simulink model "ANFISgain_tuning_simulink"  (R2024b)
settings: Solver=FixedStepAuto  StartTime=0.0  StopTime=1000  FixedStep=0.015  RelTol=1e-3
undefined symbols (not defined in the file or in its folder): sigbuilder_block, w_0
libraries: fuzblock x2, slpidlib x1, cstblocks x1
settings Model: Creator=bavejr  LastModifiedBy=lenovo pc
settings DebuggingCC: UnconnectedInputMsg=warning  UnconnectedOutputMsg=warning  UnconnectedLineMsg=warning
settings ModelReferenceCC: EnableRefExpFcnMdlSchedulingChecks=on
settings RTWCC: GPUComputeCapability=3.5  DLArmComputeVersion=19.05

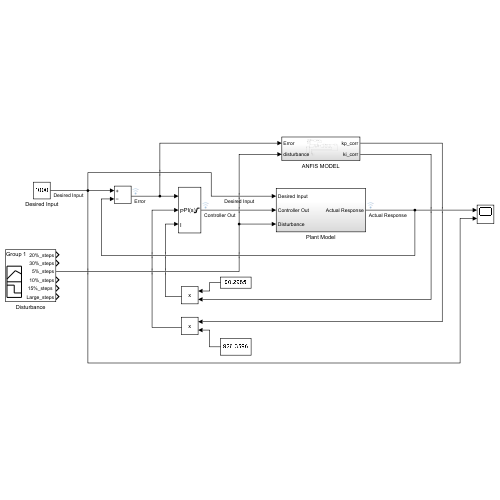
[thumbnail: Simulink's stored preview of the top-level diagram]
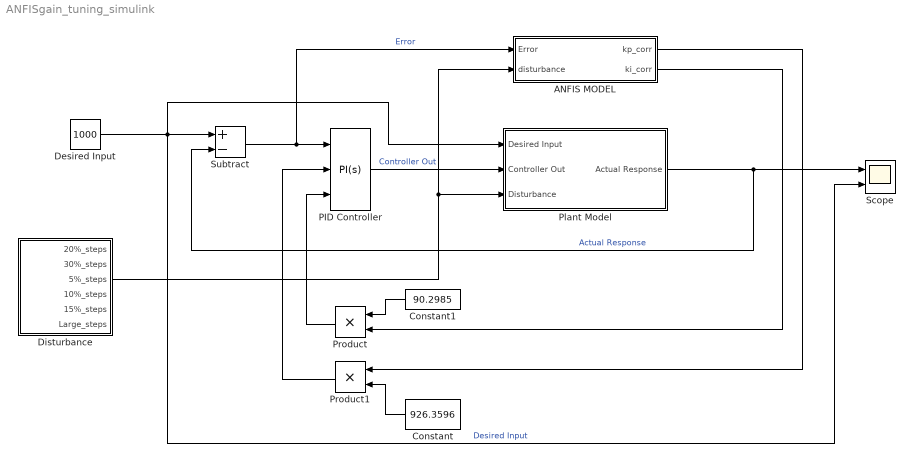
== system ANFISgain_tuning_simulink ==
  ANFIS MODEL : Subsystem
  Constant : Constant  Value=926.3596
  Constant1 : Constant  Value=90.2985
  Desired Input : Constant  Value=1000
  Disturbance : Subsystem  Tag=STV Subsys  LoadFcn=sigbuilder_block('load');  StartFcn=sigbuilder_block('start');  StopFcn=sigbuilder_block('stop');  ClipboardFcn=sigbuilder_block('clipboard');  mask(Sigbuilder block){tuvar=[0:10]}
      mask help: Simulink:masks:SigbuilderBlock_MD
      mask init:
      | if ~strcmp(get_param(bdroot(gcbh),'SimulationStatus'),'stopped') tuvar = sigbuilder_block('maskInit'); end
      settings: CopyFcn=sigbuilder_block('copy');  DeleteFcn=sigbuilder_block('delete');  ModelCloseFcn=sigbuilder_block('modelClose');  PreSaveFcn=sigbuilder_block('preSave');  PauseFcn=sigbuilder_block('pause');  ContinueFcn=sigbuilder_block('continue');  NameChangeFcn=sigbuilder_block('namechange');  OpenFcn=sigbuilder_block('open',[5.5 5.5 949 474.5 ]);  CloseFcn=sigbuilder_block('close');
      mask Display: plot(0, 0, 100, 100,[2, 2, 32, 32, 2], [68, 8, 8, 68, 68],[32, 2], [38, 38], [32, 19, 2],[53, 60, 44], [32, 17, 17, 2],[16, 16, 31, 31]);txt = getActiveGroup(gcbh);text(2, 100, txt,'verticalAlignment', 'top');
  PID Controller : slpidlib/PID Controller  Controller=PI  Form=Parallel  TimeDomain=Continuous-time  UseExternalTs=off  SampleTime=-1  IntegratorMethod=Forward Euler  FilterMethod=Forward Euler  ControllerParametersSource=external  P=8  I=2  UseKiTs=off  D=0  UseExternalDerivativeSource=off  N=100  UseFilter=on  TunerSelectOption=Frequency Response Based  InitialConditionSource=internal  InitialConditionForIntegrator=0.2  InitialConditionForFilter=0  DifferentiatorICPrevScaledInput=0  ExternalReset=none  TrackingMode=off  Kt=1  LimitOutput=on  SatLimitsSource=internal  UpperSaturationLimit=inf  LowerSaturationLimit=-inf  LinearizeAsGain=on  AntiWindupMode=back-calculation  Kb=0.0975  LimitIntegrator=off  UpperIntegratorSaturationLimit=inf  LowerIntegratorSaturationLimit=-inf  POutMin=[]  POutMax=[]  IOutMin=[]  IOutMax=[]  DOutMin=[]  DOutMax=[]  NOutMin=[]  NOutMax=[]  SumOutMin=[]  SumOutMax=[]  SaturationOutMin=[]  SaturationOutMax=[]  PParamMin=[]  PParamMax=[]  IParamMin=[]  IParamMax=[]  DParamMin=[]  DParamMax=[]  NParamMin=[]  NParamMax=[]  KbParamMin=[]  KbParamMax=[]  KtParamMin=[]  KtParamMax=[]  KbOutMin=[]  KbOutMax=[]  KtOutMin=[]  KtOutMax=[]  IntegratorOutMin=[]  IntegratorOutMax=[]  FilterOutMin=[]  FilterOutMax=[]  SumI1OutMin=[]  SumI1OutMax=[]  SumI2OutMin=[]  SumI2OutMax=[]  SumI3OutMin=[]  SumI3OutMax=[]  SumI4OutMin=[]  SumI4OutMax=[]  SumDOutMin=[]  SumDOutMax=[]  DifferentiatorOutMin=[]  DifferentiatorOutMax=[]  FilterDiffOutCoefMin=[]  FilterDiffOutCoefMax=[]  ReciprocalOutMin=[]  ReciprocalOutMax=[]  SumDenOutMin=[]  SumDenOutMax=[]  SumNumOutMin=[]  SumNumOutMax=[]  DivideOutMin=[]  DivideOutMax=[]  UdiffTsProdOutMin=[]  UdiffTsProdOutMax=[]  NTsProdOutMin=[]  NTsProdOutMax=[]  UintegralTsProdOutMin=[]  UintegralTsProdOutMax=[]  UngainTsProdOutMin=[]  UngainTsProdOutMax=[]  ClampingZeroOutDataTypeStr=Inherit: Inherit via back propagation  ClampingZeroOutMin=[]  ClampingZeroOutMax=[]  FilterDenConstantOutDataTypeStr=Inherit: Inherit via back propagation  FilterDenConstantOutMin=[]  FilterDenConstantOutMax=[]  PCopyOutDataTypeStr=Inherit: Inherit via back propagation  PCopyOutMin=[]  PCopyOutMax=[]  NCopyOutDataTypeStr=Inherit: Inherit via back propagation  NCopyOutMin=[]  NCopyOutMax=[]  IntegratorContinuousStateAttributes=''  IntegratorStateMustResolveToSignalObject=off  IntegratorRTWStateStorageClass=Auto  FilterContinuousStateAttributes=''  FilterStateMustResolveToSignalObject=off  FilterRTWStateStorageClass=Auto  ParallelPVariant=ExternalParameters  IdealPVariant=Disabled  IVariant=ExternalParameters  DVariant=Disabled  IntegratorVariant=Continuous  SatVariant=Enabled  AWVariant=BackCalculation  PCopyVariant=Disabled  TRVariant=Disabled  FdbkBlocksVariant=Forward  IdealPFdbkVariant=Disabled  SatFdbkVariant=Disabled  DerivativeFilterVariant=Disabled  NVariant=Disabled  NCopyVariant=Disabled_SignalSpec  FilterICVariant=Disabled  IntegratorICVariant=InternalICs  ExternalResetVariant=Disabled  TRSumVariant=Passthrough  SumFdbkVariant=Disabled  SumVariant=Sum_PI  TsampFilterVariant=InternalTs  TsampNgainVariant=Passthrough  TsampIntegralVariant=Disabled_SignalSpec  ExternalSaturationOutDataTypeStr=Inherit: Same as second input  DerivativeSourceVariant=Disabled  PreIntVariant=InternalPreInt
  Plant Model : Subsystem
  Product : Product
  Product1 : Product
  Scope : Scope  NumInputPorts=2
  Subtract : Sum  Inputs=+-
  wires:
  PID Controller/1 -> Plant Model/2(Controller Out)  "Controller Out"
  Plant Model/1(Actual Response) -> Subtract/2, Scope/1  "Actual Response"
  Subtract/1 -> ANFIS MODEL/1(Error), PID Controller/1  "Error"
  Desired Input/1 -> Scope/2, Plant Model/1(Desired Input), Subtract/1  "Desired Input"
  Disturbance/3(5%_steps) -> ANFIS MODEL/2(disturbance), Plant Model/3("Disturbance ")
  Constant1/1 -> Product/1
  Constant/1 -> Product1/2
  ANFIS MODEL/2(ki_corr) -> Product/2
  ANFIS MODEL/1(kp_corr) -> Product1/1
  Product/1 -> PID Controller/3
  Product1/1 -> PID Controller/2

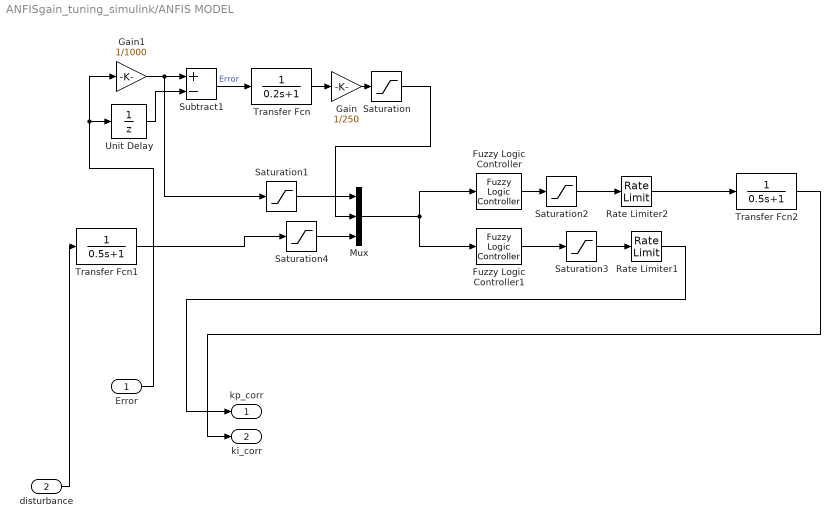
== system ANFISgain_tuning_simulink/ANFIS MODEL ==
  Error : Inport
  disturbance : Inport  Port=2
  Fuzzy Logic Controller : fuzblock/Fuzzy Logic  Controller  FIS=Ki_Model03  OutputSampleNumber=101  DataType=double  FuzzifiedInputs=off  RuleFiringStrengths=off  RuleOutputs=off  AggregatedOutputs=off  SimulateUsing=Interpreted execution  OutOfRangeInputValueMessage=warning  NoRuleFiredMessage=warning  EmptyOutputFuzzySetMessage=warning
  Fuzzy Logic Controller1 : fuzblock/Fuzzy Logic  Controller  FIS=Kp_Model03  OutputSampleNumber=101  DataType=double  FuzzifiedInputs=off  RuleFiringStrengths=off  RuleOutputs=off  AggregatedOutputs=off  SimulateUsing=Interpreted execution  OutOfRangeInputValueMessage=warning  NoRuleFiredMessage=warning  EmptyOutputFuzzySetMessage=warning
  Gain : Gain  Gain=1/250
  Gain1 : Gain  Gain=1/1000
  Mux : Mux  Inputs=3
  Rate Limiter1 : RateLimiter  RisingSlewLimit=0.02  FallingSlewLimit=-0.02  SampleTimeMode=inherited
  Rate Limiter2 : RateLimiter  RisingSlewLimit=0.005  FallingSlewLimit=-0.005  SampleTimeMode=inherited
  Saturation : Saturate  UpperLimit=1  LowerLimit=-1
  Saturation1 : Saturate  UpperLimit=1  LowerLimit=-1
  Saturation2 : Saturate  UpperLimit=2  LowerLimit=0.5
  Saturation3 : Saturate  UpperLimit=2  LowerLimit=0.5
  Saturation4 : Saturate  UpperLimit=1  LowerLimit=0
  Subtract1 : Sum  Inputs=+-
  Transfer Fcn : TransferFcn  Denominator=[0.2 1]
  Transfer Fcn1 : TransferFcn  Denominator=[0.5 1]
  Transfer Fcn2 : TransferFcn  Denominator=[0.5 1]
  Unit Delay : UnitDelay  SampleTime=0.015  HasFrameUpgradeWarning=on
  kp_corr : Outport
  ki_corr : Outport  Port=2
  wires:
  Gain/1 -> Saturation/1
  Saturation1/1 -> Mux/1
  Subtract1/1 -> Transfer Fcn/1  "Error"
  Saturation/1 -> Mux/2
  Transfer Fcn/1 -> Gain/1
  Saturation4/1 -> Mux/3
  Saturation2/1 -> Rate Limiter2/1
  Fuzzy Logic Controller1/1 -> Saturation3/1
  Rate Limiter2/1 -> Transfer Fcn2/1
  Unit Delay/1 -> Subtract1/2
  Error/1 -> Unit Delay/1, Gain1/1
  Saturation3/1 -> Rate Limiter1/1
  Transfer Fcn1/1 -> Saturation4/1
  Fuzzy Logic Controller/1 -> Saturation2/1
  Gain1/1 -> Saturation1/1, Subtract1/1
  Mux/1 -> Fuzzy Logic Controller/1, Fuzzy Logic Controller1/1
  disturbance/1 -> Transfer Fcn1/1
  Transfer Fcn2/1 -> ki_corr/1
  Rate Limiter1/1 -> kp_corr/1

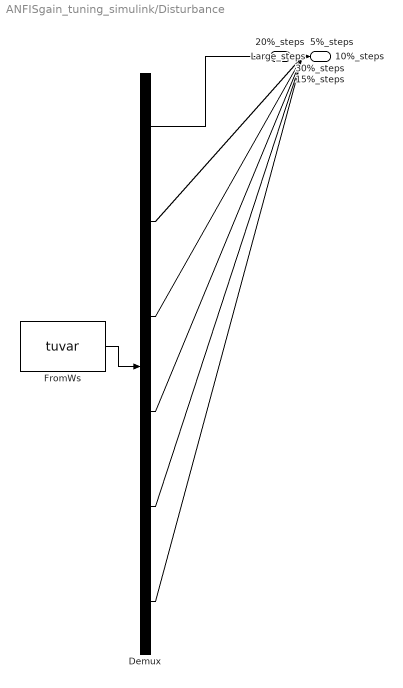
== system ANFISgain_tuning_simulink/Disturbance ==
  Demux : Demux  Tag=STV Demux  Outputs=6
      settings: DisplayOption=none
  FromWs : FromWorkspace  Tag=STV FromWs  VariableName=tuvar
      SigBuilderData=|
      | common.afterFinalStr = 'Extrapolate'
      | common.sampleTime = 0
      | dataSet.timeRange = [0 1000]
      | dataSet.name = 'Group 1'
      | sbobj.Groups.Name = 'Group 1'
      | sbobj.Groups.Signals(1).Name = '20%_steps'
      | sbobj.Groups.Signals(1).XData = [0 100 100 200 200 300 300 400 400 500 500 600 600 700 700 800 800 900 900 1000]
      | sbobj.Groups.Signals(1).YData = [0.2 0.2 0.4 0.4 0.6 0.6 0.8 0.8 1 1 0.8 0.8 0.6 0.6 0.4 0.4 0.2 0.2 0 0]
      | sbobj.Groups.Signals(2).Name = '30%_steps'
      | sbobj.Groups.Signals(2).XData = [0 120 120 240 240 360 360 480 480 600 600 720 720 840 840 960 960 1000]
      | sbobj.Groups.Signals(2).YData = [0 0 0.3 0.3 0.6 0.6 0.9 0.9 1 1 0.9 0.9 0.6 0.6 0.3 0.3 0 0]
      | sbobj.Groups.Signals(3).Name = '5%_steps'
      | sbobj.Groups.Signals(3).XData = [0 20 20 40 40 60 60 80 80 100 100 120 120 140 140 160 160 180 180 200 200 220 220 240 240 260 260 280 280 300 300 320 320 340 340 360 360 380 380 440 440 460 460 480 480 500 500 520 520 540 540 560 560 580 580 600 600 620 620 640 640 660 660 680 680 700 700 720 720 740 740 760 760 780 780 800 800 1000]
      | sbobj.Groups.Signals(3).YData = [0 0.01 0.07 0.07 0.12 0.1 0.15 0.15 0.2 0.2 0.25 0.25 0.3 0.3 0.35 0.35 0.4 0.4 0.45 0.45 0.5 0.5 0.55 0.55 0.6 0.6 0.65 0.65 0.7 0.7 0.75 0.75 0.8 0.8 0.85 0.85 0.9 0.9 0.95 0.95 0.9 0.9 0.85 0.85 0.8 0.8 0.75 0.75 0.7 0.7 0.65 0.65 0.6 0.6 0.55 0.55 0.5 0.5 0.45 0.45 0.4 0.4 0.35 0.35 0.3 0.3 0.25 0.25 0.2 0.2 0.15 0.15 0.1 0.1 0.05 0.05 0 0]
      | sbobj.Groups.Signals(4).Name = '10%_steps'
      | sbobj.Groups.Signals(4).XData = [0 50 50 100 100 150 150 200 200 250 250 300 300 350 350 400 400 450 450 500 500 550 550 600 600 650 650 700 700 750 750 800 800 850 850 900 900 950 950 1000]
      | sbobj.Groups.Signals(4).YData = [0 0 0.2 0.2 0.3 0.3 0.4 0.4 0.5 0.5 0.6 0.6 0.7 0.7 0.8 0.8 0.9 0.9 1 1 0.9 0.9 0.8 0.8 0.7 0.7 0.6 0.6 0.5 0.5 0.4 0.4 0.3 0.3 0.2 0.2 0.1 0.1 0.035 0.03]
      | sbobj.Groups.Signals(5).Name = '15%_steps '
      | sbobj.Groups.Signals(5).XData = [0 75 75 150 150 225 225 300 300 375 375 450 450 525 525 600 600 675 675 750 750 825 825 900 900 975 975 1000]
      | sbobj.Groups.Signals(5).YData = [0.15 0.15 0.3 0.3 0.45 0.45 0.6 0.6 0.75 0.75 0.9 0.9 1 1 0.9 0.9 0.75 0.75 0.6 0.6 0.45 0.45 0.3 0.3 0.15 0.15 0 0]
      | sbobj.Groups.Signals(6).Name = 'Large_steps'
      | sbobj.Groups.Signals(6).XData = [0 400 400 1000]
      | sbobj.Groups.Signals(6).YData = [0.9 0.9 0.2 0.2]
      | sbobj.Groups.TimeRange = [0 1000]
  20%_steps : Outport  Tag=STV Outport
  30%_steps : Outport  Tag=STV Outport  Port=2
  5%_steps : Outport  Tag=STV Outport  Port=3
  10%_steps : Outport  Tag=STV Outport  Port=4
  "15%_steps " : Outport  Tag=STV Outport  Port=5
  Large_steps : Outport  Tag=STV Outport  Port=6
  wires:
  FromWs/1 -> Demux/1
  Demux/1 -> 20%_steps/1
  Demux/2 -> 30%_steps/1
  Demux/3 -> 5%_steps/1
  Demux/4 -> 10%_steps/1
  Demux/5 -> "15%_steps "/1
  Demux/6 -> Large_steps/1

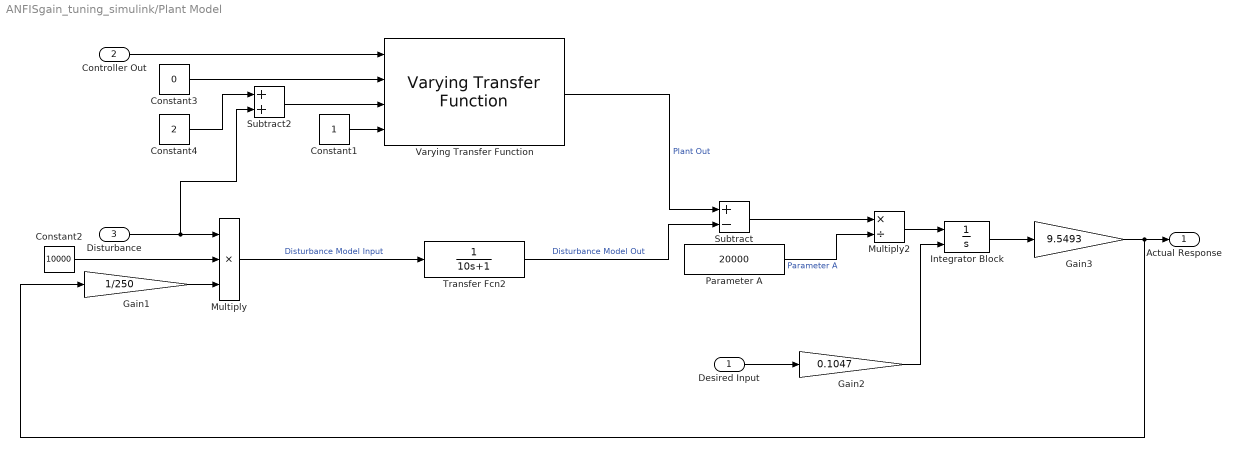
== system ANFISgain_tuning_simulink/Plant Model ==
  Desired Input : Inport
  Controller Out : Inport  Port=2
  "Disturbance " : Inport  Port=3
  Constant1 : Constant
  Constant2 : Constant  Value=10000  OutDataTypeStr=double
  Constant3 : Constant  Value=0
  Constant4 : Constant  Value=2
  Gain1 : Gain  Gain=1/250
  Gain2 : Gain  Gain=0.1047
  Gain3 : Gain  Gain=9.5493
  Integrator Block : Integrator  InitialConditionSource=external  InitialCondition=w_0  LimitOutput=on  UpperSaturationLimit=32000  LowerSaturationLimit=0
  Multiply : Product  Inputs=3  InputSameDT=on  RndMeth=Zero  SaturateOnIntegerOverflow=on  OutDataTypeStr=Inherit: Same as first input
  Multiply2 : Product  Inputs=*/
  Parameter A : Constant  Value=20000
  Subtract : Sum  Inputs=+-
  Subtract2 : Sum
  Transfer Fcn2 : TransferFcn  Denominator=[10 1]
  Varying Transfer Function : cstblocks/Linear Parameter Varying/Varying Transfer Function  N=1  Feedthrough=on
  Actual Response : Outport
  wires:
  Subtract/1 -> Multiply2/1
  Multiply2/1 -> Integrator Block/1
  Integrator Block/1 -> Gain3/1
  Desired Input/1 -> Gain2/1
  Gain2/1 -> Integrator Block/2
  Controller Out/1 -> Varying Transfer Function/1
  Gain3/1 -> Gain1/1, Actual Response/1
  Constant2/1 -> Multiply/2
  Multiply/1 -> Transfer Fcn2/1  "Disturbance Model Input"
  "Disturbance "/1 -> Subtract2/2, Multiply/1
  Transfer Fcn2/1 -> Subtract/2  "Disturbance Model Out"
  Varying Transfer Function/1 -> Subtract/1  "Plant Out"
  Gain1/1 -> Multiply/3
  Parameter A/1 -> Multiply2/2  "Parameter A"
  Constant1/1 -> Varying Transfer Function/4
  Constant3/1 -> Varying Transfer Function/2
  Subtract2/1 -> Varying Transfer Function/3
  Constant4/1 -> Subtract2/1
